simulink model "f"  (R2018b)
settings: Solver=FixedStepAuto  StartTime=0.0  StopTime=10.68  FixedStep=0.01  RelTol=1e-3
settings Model: Creator=yizha  LastModifiedBy=yizha

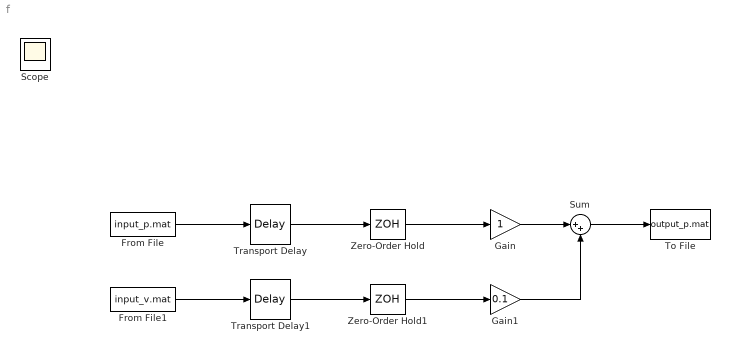
== system f ==
  From File : FromFile  FileName=input_p.mat  SampleTime=0
  From File1 : FromFile  FileName=input_v.mat  SampleTime=0
  Gain : Gain
  Gain1 : Gain  Gain=0.1
  Sum : Sum  Inputs=|++
  To File : ToFile  Filename=output_p.mat
  Transport Delay : TransportDelay  DelayTime=0.1
  Transport Delay1 : TransportDelay  DelayTime=0.1
  Zero-Order Hold : ZeroOrderHold  SampleTime=0.1
  Zero-Order Hold1 : ZeroOrderHold  SampleTime=0.1
  Scope : Scope
  wires:
  From File/1 -> Transport Delay/1
  Zero-Order Hold/1 -> Gain/1
  Transport Delay/1 -> Zero-Order Hold/1
  Transport Delay1/1 -> Zero-Order Hold1/1
  Zero-Order Hold1/1 -> Gain1/1
  From File1/1 -> Transport Delay1/1
  Gain/1 -> Sum/1
  Sum/1 -> To File/1
  Gain1/1 -> Sum/2
